simulink subsystem "Inputs_MotorDriveUnit_Drive_refsub"  (R2025a)
settings: Solver=VariableStepAuto  StartTime=0.0  StopTime=10.0  RelTol=1e-3
libraries: simulink x1
settings Model: Creator=isaacito  LastModifiedBy=isaacito

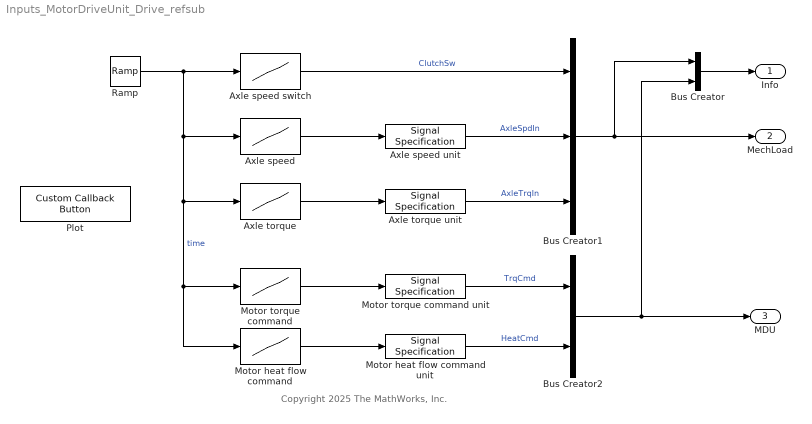
== system Inputs_MotorDriveUnit_Drive_refsub ==
  note: Copyright 2025 The MathWorks, Inc.
  Axle speed : Lookup_n-D  NumberOfTableDimensions=1  BreakpointsForDimension1=[0; 0.5; 1]  Table=[0; 0; 0]  InterpMethod=Akima spline  InternalRulePriority=Speed  RndMeth=Simplest
  Axle speed switch : Lookup_n-D  NumberOfTableDimensions=1  BreakpointsForDimension1=[0, 1]  Table=[0, 0]  InterpMethod=Flat  InternalRulePriority=Speed  RndMeth=Simplest
  Axle speed unit : SignalSpecification  Unit=rpm
  Axle torque : Lookup_n-D  NumberOfTableDimensions=1  BreakpointsForDimension1=[0; 10; 20; 21; 30.5; 40]  Table=[0; 0; 0; -10; -10; -10]  InterpMethod=Akima spline  InternalRulePriority=Speed  RndMeth=Simplest
  Axle torque unit : SignalSpecification  Unit=N*m
  Bus Creator : BusCreator  Inputs=2
  Bus Creator1 : BusCreator  Inputs=3
  Bus Creator2 : BusCreator  Inputs=2
  Motor heat flow command : Lookup_n-D  NumberOfTableDimensions=1  BreakpointsForDimension1=[0; 25; 50; 60; 130; 200; 250; 275; 300]  Table=[0; 0; 0; -2000; -2000; -2000; -12000; -12000; -12000]  InterpMethod=Akima spline  InternalRulePriority=Speed  RndMeth=Simplest
  Motor heat flow command unit : SignalSpecification  Unit=W
  Motor torque command : Lookup_n-D  NumberOfTableDimensions=1  BreakpointsForDimension1=[0; 5; 10; 60; 80; 100; 105; 152.5; 200; 205; 252.5; 300]  Table=[0; 0; 0; -300; -300; -300; 200; 200; 200; 250; 250; 250]  InterpMethod=Akima spline  InternalRulePriority=Speed  RndMeth=Simplest
  Motor torque command unit : SignalSpecification  Unit=N*m
  Plot : CustomCallbackButton  Configuration="{\"components\":[{\"name\":\"BackgroundImageComponent\",\"settings\":{\"image\":{\"size\":[0,0],\"src\":\"default\",\"srcOrientation\":\"Right\"},\"position\":[0,0,1,1]}},{\"name\":\"ButtonStateComponent\",\"settings\":{\"buttonType\":\"momentary\",\"clickFcn\":\"% Specify blocks to sort plot order.\\nblocks = [\\n  \\\"Axle speed switch\\\"\\n  \\\"Axle speed\\\"\\n  \\\"Axle torque\\\"\\n  \\\"Motor torque command\\\"\\n  \\\"Motor heat flow command\\\"\\n];\\nModelTool1.plotLookupTable1DBlocks(gcs, Blocks=blocks, DivisionType=\\\"InterpolationInterval\\\", InterpolationInterval=0.1)\",\"onValue\":1,\"position\":[0,0,1,1],\"pressDelay\":\"500\",\"pressFcn\":\"\",\"repeatInterval\":\"0\",\"states\":[{\"horizontalAlignment\":\"center\",\"image\":{\"position\":[0,0,1,1],\"size\":[1,1],\"src\":\"default\",\"srcOrientation\":\"Right\"},\"label\":{\"color\":[0.01176470588,0.01176470588,0.01176470588,1],\"icon\":{\"size\":[0,0],\"src\":\"default\",\"srcOrientation\":\"Right\"},\"iconOffset\":0,\"iconPlacement\":\"left\",\"opacity\":1,\"show\":true,\"text\":{\"content\":\"Lookup tables\",\"font\":\"Helvetica\"}},\"labelOffset\":[0,0],\"verticalAlignment\":\"middle\"},{\"horizontalAlignment\":\"center\",\"image\":{\"position\":[0,0,1,1],\"size\":[1,1],\"src\":\"default\",\"srcOrientation\":\"Right\"},\"label\":{\"color\":[0.01176470588,0.01176470588,0.01176470588,1],\"icon\":{\"size\":[0,0],\"src\":\"default\",\"srcOrientation\":\"Right\"},\"iconOffset\":0,\"iconPlacement\":\"left\",\"opacity\":1,\"show\":true,\"text\":{\"content\":\"Lookup tables\",\"font\":\"Helvetica\"}},\"labelOffset\":[0,0],\"verticalAlignment\":\"middle\"},{\"horizontalAlignment\":\"center\",\"image\":{\"position\":[0,0,1,1],\"size\":[1,1],\"src\":\"default\",\"srcOrientation\":\"Right\"},\"label\":{\"color\":[0.01176470588,0.01176470588,0.01176470588,1],\"icon\":{\"size\":[0,0],\"src\":\"default\",\"srcOrientation\":\"Right\"},\"iconOffset\":0,\"iconPlacement\":\"left\",\"opacity\":1,\"show\":true,\"text\":{\"content\":\"Lookup tables\",\"font\":\"Helvetica\"}},\"labelOffset\":[0,0],\"verticalAlignment\":\"middle\"},{\"horizontalAlignment\":\"center\",\"image\":{\"position\":[0,0,1,1],\"size\":[1,1],\"src\":\"default\",\"srcOrientation\":\"Right\"},\"label\":{\"color\":[0.01176470588,0.01176470588,0.01176470588,1],\"icon\":{\"size\":[0,0],\"src\":\"default\",\"srcOrientation\":\"Right\"},\"iconOffset\":0,\"iconPlacement\":\"left\",\"opacity\":1,\"show\":true,\"text\":{\"content\":\"Lookup tables\",\"font\":\"Helvetica\"}},\"labelOffset\":[0,0],\"verticalAlignment\":\"middle\"}]}},{\"name\":\"ForegroundImageComponent\",\"settings\":{\"image\":{\"size\":[0,0],\"src\":\"default\",\"srcOrientation\":\"Right\"},\"isForeground\":1,\"position\":[0,0,1,1]}}],\"derived\":{\"blockParameters\":{\"AutoActivate\":true,\"ButtonText\":\"Lookup tables\",\"ButtonType\":\"Momentary\",\"ClickFcn\":\"% Specify blocks to sort plot order.\\nblocks = [\\n  \\\"Axle speed switch\\\"\\n  \\\"Axle speed\\\"\\n  \\\"Axle torque\\\"\\n  \\\"Motor torque command\\\"\\n  \\\"Motor heat flow command\\\"\\n];\\nModelTool1.plotLookupTable1DBlocks(gcs, Blocks=blocks, DivisionType=\\\"InterpolationInterval\\\", InterpolationInterval=0.1)\",\"OnValue\":1,\"PressDelay\":\"500\",\"PressFcn\":\"\",\"RepeatInterval\":\"0\",\"fixedAspectRatio\":\"off\"}},\"settings\":{\"BindingType\":\"standalone\",\"autoActivate\":true,\"backgroundColor\":[244,244,244,1],\"backgroundOffset\":0.2,\"backgroundOpacity\":1,\"fixedAspectRatio\":\"off\",\"foregroundColor\":[0.01176470588,0.01176470588,0.01176470588,1],\"migratedFromLegacy\":true,\"useBackgroundColor\":true,\"variant\":\"callback\",\"version\":\"R2025a\"},\"type\":\"Button\"}"  CustomBackgroundColor="{\"color\":[0.9568627451,0.9568627451,0.9568627451],\"show\":true}"
  Ramp : simulink/Sources/Ramp  slope=1  start=0  InitialOutput=0
      settings: AttributesFormatString=|
      | Slope: %<slope>
      | Start time: %<start>
      | Initial output: %<InitialOutput>
  Info : Outport
  MechLoad : Outport  Port=2
  MDU : Outport  Port=3
  wires:
  Bus Creator/1 -> Info/1
  Motor torque command unit/1 -> Bus Creator2/1  "TrqCmd"
  Axle torque unit/1 -> Bus Creator1/3  "AxleTrqIn"
  Axle speed unit/1 -> Bus Creator1/2  "AxleSpdIn"
  Motor heat flow command unit/1 -> Bus Creator2/2  "HeatCmd"
  Bus Creator2/1 -> Bus Creator/2, MDU/1
  Bus Creator1/1 -> Bus Creator/1, MechLoad/1
  Ramp/1 -> Motor heat flow command/1, Motor torque command/1, Axle torque/1, Axle speed/1, Axle speed switch/1  "time"
  Axle speed switch/1 -> Bus Creator1/1  "ClutchSw"
  Axle speed/1 -> Axle speed unit/1
  Axle torque/1 -> Axle torque unit/1
  Motor torque command/1 -> Motor torque command unit/1
  Motor heat flow command/1 -> Motor heat flow command unit/1
